simulink model "project_"  (R2018b)
settings: Solver=VariableStepAuto  StartTime=0.0  StopTime=10.0  RelTol=1e-3
libraries: sharedTrackingLibrary x2
settings Model: Creator=computer  LastModifiedBy=computer

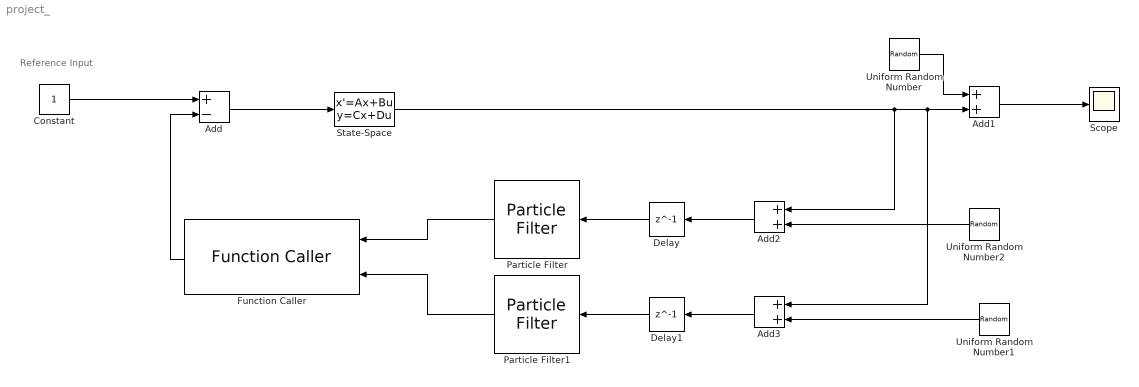
== system project_ ==
  note: Reference Input
  Add : Sum  Inputs=+-
  Add1 : Sum
  Add2 : Sum
  Add3 : Sum
  Constant : Constant
  Delay : Delay  DelayLength=1
  Delay1 : Delay  DelayLength=1
  Function Caller : FunctionCaller  FunctionPrototype=u = f(x1_dot,x2_dot)
  Particle Filter : sharedTrackingLibrary/Particle Filter  StateTransitionFcn=vdpParticleFilterStateFcn  HasStateTransitionFcnExtraArgument=0  NumberOfParticles=1000  InitialDistribution=Gaussian  InitialMean=[0; 0]  InitialCovariance=1  InitialStateBounds=[-3 3; -3 3]  InitialParticles=[]  InitialWeights=[]  CircularVariables=0  StateOrientation=Column  MeasurementLikelihoodFcn1=vdpMeasurementLikelihoodFcn  HasMeasurementEnablePort1=off  HasMeasurementFcnExtraArgument1=0  HasMeasurementEnablePort2=off  HasMeasurementFcnExtraArgument2=0  HasMeasurementEnablePort3=off  HasMeasurementFcnExtraArgument3=0  HasMeasurementEnablePort4=off  HasMeasurementFcnExtraArgument4=0  HasMeasurementEnablePort5=off  HasMeasurementFcnExtraArgument5=0  ResamplingMethod=Multinomial  TriggerMethod=Ratio  MinEffectiveParticleRatio=0.5  SamplingInterval=1  Randomness=Repeatable  Seed=0  StateEstimationMethod=Mean  OutputParticles=off  OutputWeights=off  OutputStateCovariance=off  UseCurrentEstimator=on  EnableMultirate=off  StateTransitionFcnSampleTime=1  MeasurementLikelihoodFcn1SampleTime=1  MeasurementLikelihoodFcn2SampleTime=1  MeasurementLikelihoodFcn3SampleTime=1  MeasurementLikelihoodFcn4SampleTime=1  MeasurementLikelihoodFcn5SampleTime=1  DataType=double  SampleTime=1  NumberOfMeasurements=1
      settings: SourceProductName=Control System Toolbox  SourceProductBaseCode=CT
  Particle Filter1 : sharedTrackingLibrary/Particle Filter  StateTransitionFcn=vdpParticleFilterStateFcn  HasStateTransitionFcnExtraArgument=0  NumberOfParticles=1000  InitialDistribution=Gaussian  InitialMean=[0; 0]  InitialCovariance=1  InitialStateBounds=[-3 3; -3 3]  InitialParticles=[]  InitialWeights=[]  CircularVariables=0  StateOrientation=Column  MeasurementLikelihoodFcn1=vdpMeasurementLikelihoodFcn  HasMeasurementEnablePort1=off  HasMeasurementFcnExtraArgument1=0  HasMeasurementEnablePort2=off  HasMeasurementFcnExtraArgument2=0  HasMeasurementEnablePort3=off  HasMeasurementFcnExtraArgument3=0  HasMeasurementEnablePort4=off  HasMeasurementFcnExtraArgument4=0  HasMeasurementEnablePort5=off  HasMeasurementFcnExtraArgument5=0  ResamplingMethod=Multinomial  TriggerMethod=Ratio  MinEffectiveParticleRatio=0.5  SamplingInterval=1  Randomness=Repeatable  Seed=0  StateEstimationMethod=Mean  OutputParticles=off  OutputWeights=off  OutputStateCovariance=off  UseCurrentEstimator=on  EnableMultirate=off  StateTransitionFcnSampleTime=1  MeasurementLikelihoodFcn1SampleTime=1  MeasurementLikelihoodFcn2SampleTime=1  MeasurementLikelihoodFcn3SampleTime=1  MeasurementLikelihoodFcn4SampleTime=1  MeasurementLikelihoodFcn5SampleTime=1  DataType=double  SampleTime=1  NumberOfMeasurements=1
      settings: SourceProductName=Control System Toolbox  SourceProductBaseCode=CT
  Scope : Scope
  State-Space : StateSpace  InitialCondition=0
  Uniform Random Number : UniformRandomNumber  SampleTime=0.1
  Uniform Random Number1 : UniformRandomNumber  SampleTime=0.1
  Uniform Random Number2 : UniformRandomNumber  SampleTime=0.1
  wires:
  Constant/1 -> Add/1
  Add/1 -> State-Space/1
  State-Space/1 -> Add2/1, Add3/1, Add1/2
  Function Caller/1 -> Add/2
  Particle Filter1/1 -> Function Caller/2
  Particle Filter/1 -> Function Caller/1
  Delay/1 -> Particle Filter/1
  Delay1/1 -> Particle Filter1/1
  Add2/1 -> Delay/1
  Add3/1 -> Delay1/1
  Add1/1 -> Scope/1
  Uniform Random Number/1 -> Add1/1
  Uniform Random Number1/1 -> Add3/2
  Uniform Random Number2/1 -> Add2/2
